simulink model "PIController"  (R2018b)
settings: Solver=VariableStepAuto  StartTime=0.0  StopTime=500  RelTol=1e-3
undefined symbols (not defined in the file): sigbuilder_block
libraries: VehicleMdl x1
settings Model: Creator=Lenovo  LastModifiedBy=Lenovo

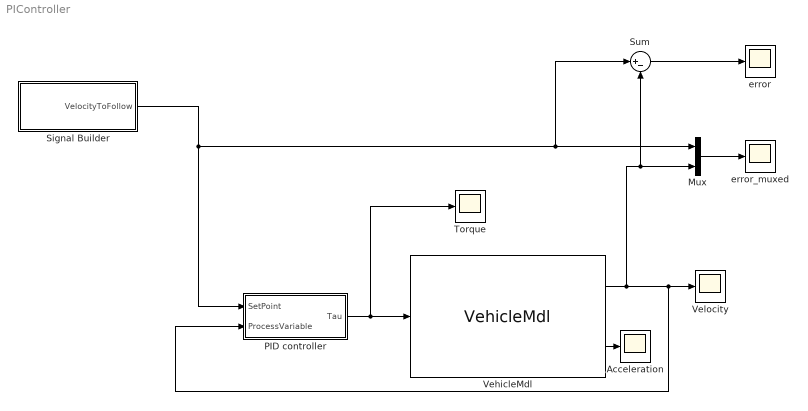
== system PIController ==
  Acceleration : Scope
  Mux : Mux  Inputs=2
  PID controller : Subsystem
  Signal Builder : Subsystem  Tag=STV Subsys  LoadFcn=sigbuilder_block('load',[0.75 0.75 718.5 340.5 ]);  StartFcn=sigbuilder_block('start');  StopFcn=sigbuilder_block('stop');  ClipboardFcn=sigbuilder_block('clipboard');  mask(Sigbuilder block){tuvar=[0:10]}
      mask help: Simulink:masks:SigbuilderBlock_MD
      mask init:
      | if ~strcmp(get_param(bdroot(gcbh),'SimulationStatus'),'stopped') tuvar = sigbuilder_block('maskInit'); end
      settings: CopyFcn=sigbuilder_block('copy');  DeleteFcn=sigbuilder_block('delete');  ModelCloseFcn=sigbuilder_block('modelClose');  PreSaveFcn=sigbuilder_block('preSave');  PauseFcn=sigbuilder_block('pause');  ContinueFcn=sigbuilder_block('continue');  NameChangeFcn=sigbuilder_block('namechange');  OpenFcn=sigbuilder_block('open',[0.75 0.75 718.5 340.5 ]);  CloseFcn=sigbuilder_block('close');
      mask Display: plot(0, 0, 100, 100,[2, 2, 32, 32, 2], [68, 8, 8, 68, 68],[32, 2], [38, 38], [32, 19, 2],[53, 60, 44], [32, 17, 17, 2],[16, 16, 31, 31]);txt = getActiveGroup(gcbh);text(2, 100, txt,'verticalAlignment', 'top');
  Sum : Sum  Inputs=|+-
  "Torque " : Scope
  VehicleMdl : VehicleMdl/VehicleMdl  v_max=42  v_min=0  a_max=3  a_min=-3
  Velocity : Scope
  error : Scope
  "error_muxed " : Scope
  wires:
  VehicleMdl/1 -> Mux/2, Sum/2, PID controller/2(ProcessVariable), Velocity/1
  VehicleMdl/2 -> Acceleration/1
  Signal Builder/1(VelocityToFollow) -> PID controller/1("SetPoint "), Sum/1, Mux/1
  Mux/1 -> "error_muxed "/1
  Sum/1 -> error/1
  PID controller/1(Tau) -> "Torque "/1, VehicleMdl/1

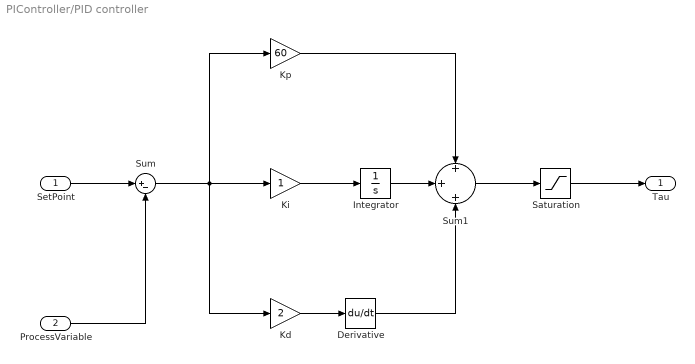
== system PIController/PID controller ==
  "SetPoint " : Inport
  ProcessVariable : Inport  Port=2
  Derivative : Derivative
  Integrator : Integrator
  "Kd " : Gain  Gain=2
  Ki : Gain
  Kp : Gain  Gain=60
  Saturation : Saturate  UpperLimit=130  LowerLimit=-130  ZeroCross=off
  Sum : Sum  Inputs=|+-
  Sum1 : Sum  Inputs=+|+|+
  Tau : Outport
  wires:
  "SetPoint "/1 -> Sum/1
  ProcessVariable/1 -> Sum/2
  Sum/1 -> Kp/1, "Kd "/1, Ki/1
  Derivative/1 -> Sum1/3
  Kp/1 -> Sum1/1
  Sum1/1 -> Saturation/1
  "Kd "/1 -> Derivative/1
  Integrator/1 -> Sum1/2
  Ki/1 -> Integrator/1
  Saturation/1 -> Tau/1

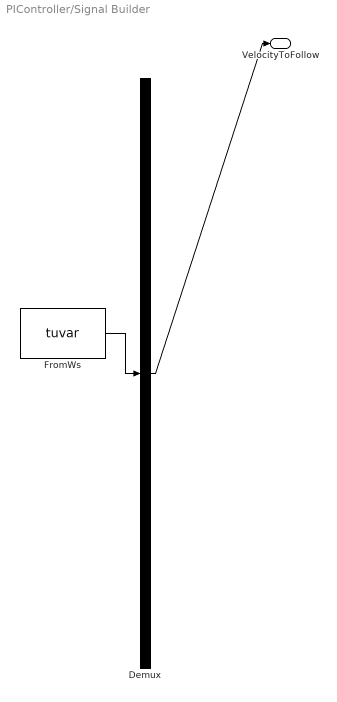
== system PIController/Signal Builder ==
  Demux : Demux  Tag=STV Demux  Outputs=1
  FromWs : FromWorkspace  Tag=STV FromWs  VariableName=tuvar  SampleTime=0
      SigBuilderData=|
      | common.afterFinalStr = 'Extrapolate'
      | common.sampleTime = 0
      | dataSet.timeRange = [0 500]
      | dataSet.name = 'Group 1'
      | sbobj.Groups.Name = 'Group 1'
      | sbobj.Groups.Signals.Name = 'VelocityToFollow'
      | sbobj.Groups.Signals.XData = [0 10 20 30 75 100 130 150 200 250 300 330 400 410 430 450 470 500]
      | sbobj.Groups.Signals.YData = [0 6 6 3 25 25 15 15 40.5 32 32 20 20 14.5 14 5 5 0]
      | sbobj.Groups.TimeRange = [0 500]
  VelocityToFollow : Outport  Tag=STV Outport
  wires:
  FromWs/1 -> Demux/1
  Demux/1 -> VelocityToFollow/1
